simulink model "DC_Motor_Control_PM"  (R2022b)
settings: Solver=ode23s  StartTime=0.0  StopTime=0.2  RelTol=1e-3  EnableMultiTasking=on
undefined symbols (not defined in the file): B, J, K, ki_curr, ki_speed, kp_curr, kp_speed, La, Ra
settings Model: Creator=matti  LastModifiedBy=Alessandro
settings SolverCC: AlgebraicLoopSolver=TrustRegion
settings DataIOCC: LimitDataPoints=on  SaveFormat=Array  ReturnWorkspaceOutputs=off
settings OptimizationCC: LifeSpan=inf
settings DebuggingCC: SolverPrmCheckMsg=warning  UnconnectedInputMsg=warning  UnconnectedOutputMsg=warning  UnconnectedLineMsg=warning  SFUnexpectedBacktrackingDiag=warning  SFNoUnconditionalDefaultTransitionDiag=warning  SFExecutionAtInitializationDiag=none  SFMachineParentedDataDiag=warning  ArithmeticOperatorsInVariantConditions=warning
settings HardwareCC: ProdBitPerPointer=32  ProdBitPerSizeT=32  ProdBitPerPtrDiffT=32  ProdLargestAtomicFloat=None  ProdIntDivRoundTo=Undefined  ProdEndianess=Unspecified  ProdWordSize=32  ProdHWDeviceType=32-bit Generic
settings ModelReferenceCC: EnableRefExpFcnMdlSchedulingChecks=on  PropagateSignalLabelsOutOfModel=off
settings SFSimCC: SimUseLocalCustomCode=off  CustomCodeUndefinedFunction=UseInterfaceOnly
settings RTWCC: RTWUseLocalCustomCode=off
settings CodeAppCC: StateflowObjectComments=on
settings GRTTargetCC: TargetLangStandard=C89/C90 (ANSI)
settings ConfigComp: CovMetricSettings=dw  CovSaveCumulativeToWorkspaceVar=on  CovSaveSingleToWorkspaceVar=on  CovExternalEMLEnable=off  CovSFcnEnable=off

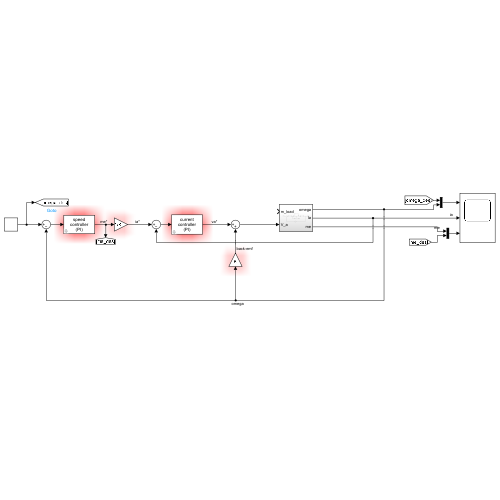
[thumbnail: Simulink's stored preview of the top-level diagram]
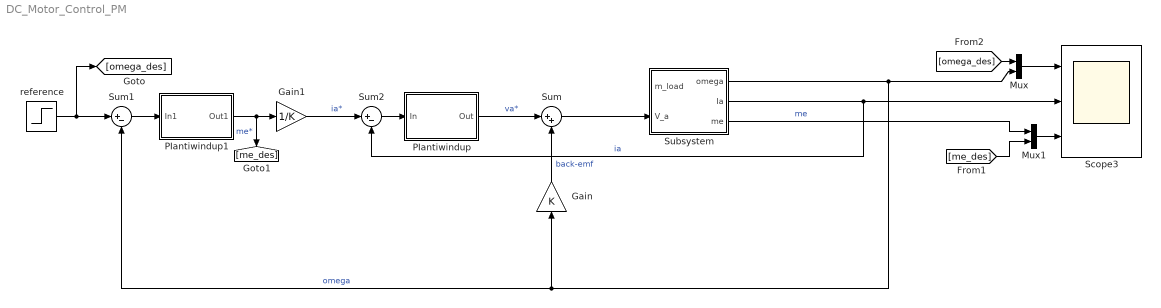
== system DC_Motor_Control_PM ==
  Gain : Gain  Gain=K
  Gain1 : Gain  Gain=1/K
  Mux : Mux  Inputs=2
  Mux1 : Mux  Inputs=2
  PIantiwindup : Subsystem  mask{Kp=kp_curr, Ki=ki_curr, sat_up=600, sat_down=-600}
      mask prompts: sat_up "Upper sat. limit"; sat_down "Lower Sat. Limit"
      mask Display: disp('current\ncontroller\n(PI)')
  PIantiwindup1 : Subsystem  mask{Kp=kp_speed, Ki=ki_speed, sat_up=1000, sat_down=-1000}
      mask prompts: sat_up "Upper sat. limit"; sat_down "Lower Sat. Limit"
      mask Display: disp('speed\ncontroller\n(PI)')
  Scope3 : Scope  NumInputPorts=3
  Subsystem : Subsystem
  Sum : Sum  Inputs=|++
  Sum1 : Sum  Inputs=|+-
  Sum2 : Sum  Inputs=|+-
  reference : Step  Time=0  After=300  SampleTime=0
  wires:
  Subsystem/1(omega) -> Sum1/2, Gain/1, Mux/2  "omega"
  PIantiwindup/1(Out) -> Sum/1  "va*"
  Sum2/1 -> PIantiwindup/1(In)
  PIantiwindup1/1(Out1) -> Gain1/1, [me_des]  "me*"
  reference/1 -> Sum1/1, [omega_des]
  Sum1/1 -> PIantiwindup1/1(In1)
  Subsystem/2(Ia) -> Sum2/2, Scope3/2  "ia"
  Subsystem/3(me) -> Mux1/1  "me"
  Gain/1 -> Sum/2  "back-emf"
  Gain1/1 -> Sum2/1  "ia*"
  Mux/1 -> Scope3/1
  [me_des] -> Mux1/2
  Mux1/1 -> Scope3/3
  [omega_des] -> Mux/1
  Sum/1 -> Subsystem/2(V_a)

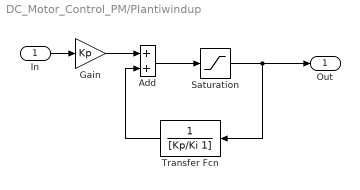
== system DC_Motor_Control_PM/PIantiwindup ==
  In : Inport
  Add : Sum
  Gain : Gain  Gain=Kp
  Saturation : Saturate  UpperLimit=sat_up  LowerLimit=sat_down
  Transfer Fcn : TransferFcn  Denominator=[Kp/Ki 1]
  Out : Outport  VectorParamsAs1DForOutWhenUnconnected=off
  wires:
  Saturation/1 -> Out/1, Transfer Fcn/1
  In/1 -> Gain/1
  Gain/1 -> Add/1
  Add/1 -> Saturation/1
  Transfer Fcn/1 -> Add/2

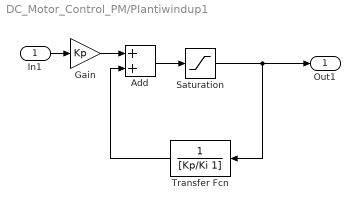
== system DC_Motor_Control_PM/PIantiwindup1 ==
  In1 : Inport
  Add : Sum
  Gain : Gain  Gain=Kp
  Saturation : Saturate  UpperLimit=sat_up  LowerLimit=sat_down
  Transfer Fcn : TransferFcn  Denominator=[Kp/Ki 1]
  Out1 : Outport  VectorParamsAs1DForOutWhenUnconnected=off
  wires:
  Transfer Fcn/1 -> Add/2
  Add/1 -> Saturation/1
  Gain/1 -> Add/1
  In1/1 -> Gain/1
  Saturation/1 -> Transfer Fcn/1, Out1/1

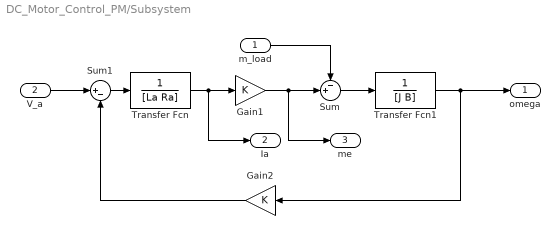
== system DC_Motor_Control_PM/Subsystem ==
  m_load : Inport
  V_a : Inport  Port=2
  Gain1 : Gain  Gain=K
  Gain2 : Gain  Gain=K
  Sum : Sum  Inputs=-+|
  Sum1 : Sum  Inputs=|+-
  Transfer Fcn : TransferFcn  Denominator=[La Ra]
  Transfer Fcn1 : TransferFcn  Denominator=[J B]
  omega : Outport  VectorParamsAs1DForOutWhenUnconnected=off
  Ia : Outport  Port=2  VectorParamsAs1DForOutWhenUnconnected=off
  me : Outport  Port=3  VectorParamsAs1DForOutWhenUnconnected=off
  wires:
  m_load/1 -> Sum/1
  Gain2/1 -> Sum1/2
  Sum1/1 -> Transfer Fcn/1
  Gain1/1 -> me/1, Sum/2
  Transfer Fcn/1 -> Ia/1, Gain1/1
  Transfer Fcn1/1 -> omega/1, Gain2/1
  Sum/1 -> Transfer Fcn1/1
  V_a/1 -> Sum1/1
